simulink model "test"  (R2024b)
settings: Solver=ode4  StartTime=0.0  StopTime=2000  FixedStep=0.01  RelTol=1e-3
values from neighbouring files (symbols this model uses):
  g0 = 9.81    [llm_scenarios_case2.m]
  I_total = 0.5*(I_total + I_total.')    [total_inertia.m]    (also in total_inertia_backup.m = I_total + I_transformed)
undefined symbols (not defined in the file or in its folder): f_plant, GEOSAT, LLM, Mi, sigma_pos, sigma_vel, ST, Uoff, Uon
libraries: simulink x13, sharedTrackingLibrary x1
settings Model: Creator=simon  LastModifiedBy=simon
settings OptimizationCC: DefaultParameterBehavior=Inlined  EnhancedBackFolding=on  PassReuseOutputArgsAs=Individual arguments  ZeroExternalMemoryAtStartup=off  ZeroInternalMemoryAtStartup=off  MaxStackSize=64  OptimizeBlockOrder=speed  DifferentSizesBufferReuse=on  OptimizationCustomize=off  EfficientTunableParamExpr=on
settings DebuggingCC: ParameterTunabilityLossMsg=error
settings SFSimCC: MATLABDynamicMemAlloc=off
settings RTWCC: Description=Embedded Coder  SystemTargetFile=ert.tlc  HardwareBoard=Robot Operating System 2 (ROS 2)  TLCOptions="-aInlineSetEventsForThisBaseRateFcn=TLC_FALSE -aSuppressMultiTaskScheduler=TLC_FALSE  -aRateBasedStepFcn=0"  TemplateMakefile=ert_default_tmf  Toolchain=Colcon Tools  TargetLang=C++
settings CodeAppCC: ForceParamTrailComments=on  IgnoreCustomStorageClasses=off  OperatorAnnotations=on  SimulinkDataObjDesc=on  SFDataObjDesc=on  InsertBlockDesc=on
settings ERTTargetCC: CodeInterfacePackaging=C++ class  RootIOFormat=Structure reference

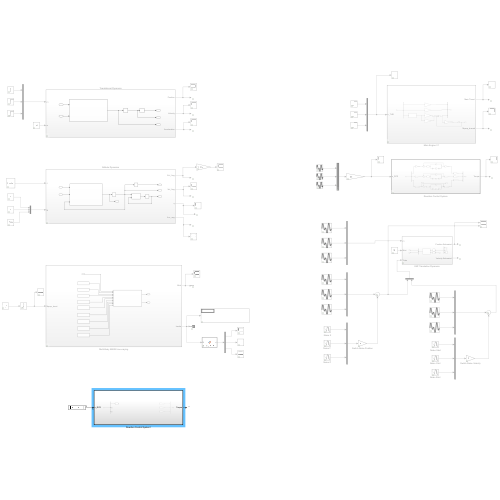
[thumbnail: Simulink's stored preview of the top-level diagram]
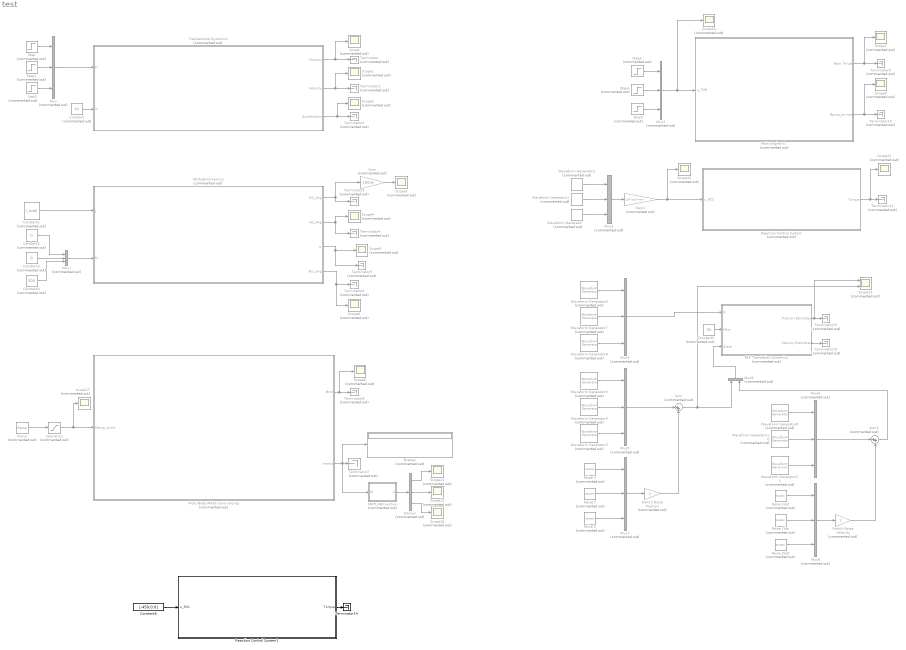
== system test ==
  " Noise X" : RandomNumber  Commented=on  Variance=sigma_pos^2  Seed=1  SampleTime=1/f_plant
  " Noise Xdot" : RandomNumber  Commented=on  Variance=sigma_vel^2  Seed=1  SampleTime=1/f_plant
  Attitude Dynamics : Subsystem  Commented=on
  Constant : Constant  Commented=on  Value=Mi
  Constant1 : Constant  Commented=on  Value=I_total
  Constant2 : Constant  Commented=on  Value=0
  Constant3 : Constant  Commented=on  Value=0
  Constant4 : Constant  Commented=on  Value=500
  Constant5 : Constant  Commented=on  Value=Mi
  Constant6 : Constant  Value=[-450;0;0]
  Demux : Demux  Commented=on  Outputs=3
  Display : Display  Commented=on
  EKF Translation Dynamics : Subsystem  Commented=on
  Gain : Gain  Commented=on  Gain=180/pi
  Gain1 : Gain  Commented=on  Gain=LLM.rcs.Fmax
  MATLAB Function : MATLAB Function  Commented=on  TreatAsAtomicUnit=on
  Main Engine V1 : Subsystem  Commented=on
  Multi-Body MASS time-varying : Subsystem  Commented=on
  Mux{,1..8} (9 alike) : Mux  Commented=on  Inputs=3
  Mux9 : Mux  Commented=on  Inputs=2
  Noise Y : RandomNumber  Commented=on  Variance=sigma_pos^2  Seed=2  SampleTime=1/f_plant
  Noise Ydot : RandomNumber  Commented=on  Variance=sigma_vel^2  Seed=2  SampleTime=1/f_plant
  Noise Z : RandomNumber  Commented=on  Variance=sigma_pos^2  Seed=3  SampleTime=1/f_plant
  Noise Zdot : RandomNumber  Commented=on  Variance=sigma_vel^2  Seed=3  SampleTime=1/f_plant
  Ramp : simulink/Sources/Ramp  Commented=on  slope=10  start=0  InitialOutput=0
  Reaction Control System : Subsystem  Commented=on  TreatAsAtomicUnit=on
  Reaction Control System1 : Subsystem  TreatAsAtomicUnit=on
  Saturation : Saturate  Commented=on  UpperLimit=0.01*LLM.propellant.mass  LowerLimit=0
  Scope{,1..12,14..17} (17 alike) : Scope  Commented=on
  Scope13 : Scope  Commented=on  NumInputPorts=2
  Step : Step  Commented=on  After=0  SampleTime=0
  Step1 : Step  Commented=on  After=0  SampleTime=0
  Step2 : Step  Commented=on  After=LLM.main_engine.Fmax  SampleTime=0
  Step3 : Step  Commented=on  Time=30  After=0.4  SampleTime=0
  Step4 : Step  Commented=on  Time=30  After=0.4  SampleTime=0
  Step5 : Step  Commented=on  Time=30  After=0.5  SampleTime=0
  Sum : Sum  Commented=on  Inputs=|++
  Sum1 : Sum  Commented=on  Inputs=|++
  Switch Noise Position : Gain  Commented=on
  Switch Noise Velocity : Gain  Commented=on
  Terminator{,1..13} (14 alike) : Terminator  Commented=on
  Terminator14 : Terminator
  Translational Dynamics : Subsystem  Commented=on
  Waveform Generator : simulink/Sources/Waveform Generator  Commented=on  OutMin=[]  OutMax=[]  OutDataTypeStr=double  SelectedSignal=1  Signals=sin('Amplitude', 1, 'Frequency', 0.3, 'Phase', 0)  BlockNames=MultiportSwitch_2c032cfd7e664ef  SampleTime=0.1
  Waveform Generator1 : simulink/Sources/Waveform Generator  Commented=on  OutMin=[]  OutMax=[]  OutDataTypeStr=double  SelectedSignal=1  Signals=sin('Amplitude', 1, 'Frequency', 0.3, 'Phase', 0)  BlockNames=MultiportSwitch_2c032cfd7e664ef  SampleTime=0.1
  Waveform Generator10 : simulink/Sources/Waveform Generator  Commented=on  OutMin=[]  OutMax=[]  OutDataTypeStr=double  SelectedSignal=1  Signals=cos(10, 1, 0)  BlockNames=MultiportSwitch_2c7686f9e0bf4b8  SampleTime=0.1
  Waveform Generator11 : simulink/Sources/Waveform Generator  Commented=on  OutMin=[]  OutMax=[]  OutDataTypeStr=double  SelectedSignal=1  Signals=cos(10, 1, 0)  BlockNames=MultiportSwitch_733c71b08a0b470  SampleTime=0.1
  Waveform Generator2 : simulink/Sources/Waveform Generator  Commented=on  OutMin=[]  OutMax=[]  OutDataTypeStr=double  SelectedSignal=1  Signals=sin('Amplitude', 1, 'Frequency', 0.3, 'Phase', 0)  BlockNames=MultiportSwitch_2c032cfd7e664ef  SampleTime=0.1
  Waveform Generator{3..8} (6 alike) : simulink/Sources/Waveform Generator  Commented=on  OutMin=[]  OutMax=[]  OutDataTypeStr=double  SelectedSignal=1  Signals=sin(10, 1, 0)  BlockNames=MultiportSwitch_61beab59be99459  SampleTime=0.1
  Waveform Generator9 : simulink/Sources/Waveform Generator  Commented=on  OutMin=[]  OutMax=[]  OutDataTypeStr=double  SelectedSignal=1  Signals=cos(10, 1, 0)  BlockNames=MultiportSwitch_701aef0e77f74ea  SampleTime=0.1
  wires:
  Mux/1 -> Translational Dynamics/1(FI)
  Constant/1 -> Translational Dynamics/2(m)
  Translational Dynamics/1(Position) -> Scope/1, Terminator/1
  Translational Dynamics/2(Velocity) -> Scope1/1, Terminator1/1
  Translational Dynamics/3(Acceleration) -> Scope2/1, Terminator2/1
  Step/1 -> Mux/1
  Step1/1 -> Mux/2
  Step2/1 -> Mux/3
  Attitude Dynamics/1(Eul_Ang) -> Gain/1, Terminator3/1
  Attitude Dynamics/2(Vel_Ang) -> Scope4/1, Terminator4/1
  Constant2/1 -> Mux1/1
  Constant3/1 -> Mux1/2
  Constant4/1 -> Mux1/3
  Mux1/1 -> Attitude Dynamics/2(M)
  Gain/1 -> Scope3/1
  Constant1/1 -> Attitude Dynamics/1(J)
  Attitude Dynamics/3(q) -> Scope5/1, Terminator5/1
  Attitude Dynamics/4(Acc_ang) -> Scope6/1, Terminator6/1
  Multi-Body MASS time-varying/1(Mtot) -> Terminator8/1, Scope8/1
  Ramp/1 -> Saturation/1
  Multi-Body MASS time-varying/2(Inertia) -> Display/1, Terminator7/1, MATLAB Function/1(M)
  Mux2/1 -> Scope10/1, Main Engine V1/1(u_THR)
  Step3/1 -> Mux2/1
  Step4/1 -> Mux2/2
  Step5/1 -> Mux2/3
  Main Engine V1/2(Mprop_burned) -> Scope9/1, Terminator10/1
  Main Engine V1/1("Main Thrust ") -> Scope7/1, Terminator9/1
  Gain1/1 -> Scope12/1, Reaction Control System/1(u_RCS)
  Reaction Control System/1(Torque) -> Scope11/1, Terminator11/1
  Waveform Generator2/1 -> Mux3/1
  Waveform Generator1/1 -> Mux3/2
  Mux3/1 -> Gain1/1
  Waveform Generator/1 -> Mux3/3
  Waveform Generator7/1 -> Mux4/2
  Waveform Generator6/1 -> Mux4/1
  Waveform Generator8/1 -> Mux4/3
  Waveform Generator3/1 -> Mux5/1
  Waveform Generator4/1 -> Mux5/2
  Waveform Generator5/1 -> Mux5/3
  Constant5/1 -> EKF Translation Dynamics/2(Mtot)
  Mux4/1 -> EKF Translation Dynamics/1(FI)
  EKF Translation Dynamics/1(Position Estimated) -> Scope13/1, Terminator12/1
  EKF Translation Dynamics/2(Velocity Estimated) -> Terminator13/1
  Waveform Generator10/1 -> Mux6/2
  Waveform Generator9/1 -> Mux6/1
  Waveform Generator11/1 -> Mux6/3
  " Noise Xdot"/1 -> Mux8/1
  Noise Y/1 -> Mux7/2
  Noise Ydot/1 -> Mux8/2
  Noise Zdot/1 -> Mux8/3
  " Noise X"/1 -> Mux7/1
  Noise Z/1 -> Mux7/3
  Mux8/1 -> Switch Noise Velocity/1
  Mux7/1 -> Switch Noise Position/1
  Mux5/1 -> Sum/1
  Switch Noise Position/1 -> Sum/2
  Mux6/1 -> Sum1/1
  Switch Noise Velocity/1 -> Sum1/2
  Sum/1 -> Mux9/1, Scope13/2
  Sum1/1 -> Mux9/2
  Mux9/1 -> EKF Translation Dynamics/3(State)
  MATLAB Function/1(d) -> Demux/1
  Demux/1 -> Scope14/1
  Demux/2 -> Scope15/1
  Demux/3 -> Scope16/1
  Saturation/1 -> Scope17/1, Multi-Body MASS time-varying/1(Mprop_burnt)
  Constant6/1 -> Reaction Control System1/1(u_RCS)
  Reaction Control System1/1(Torque) -> Terminator14/1

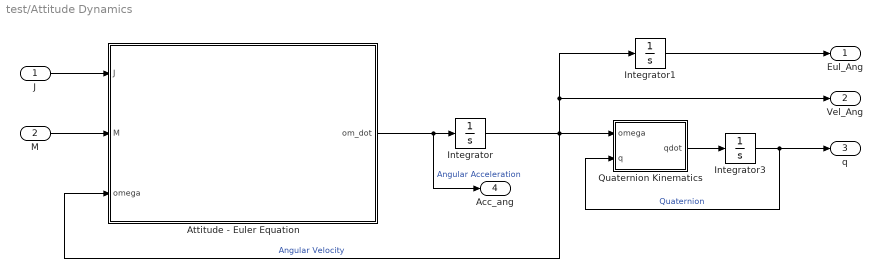
== system test/Attitude Dynamics ==
  J : Inport
  M : Inport  Port=2
  Attitude - Euler Equation : MATLAB Function  TreatAsAtomicUnit=on
  Integrator : Integrator  InitialCondition=[0;0;0]
  Integrator1 : Integrator  InitialCondition=[0;0;0]
  Integrator3 : Integrator  InitialCondition=[0;0;0;0]
  Quaternion Kinematics : MATLAB Function  TreatAsAtomicUnit=on
  Eul_Ang : Outport
  Vel_Ang : Outport  Port=2
  q : Outport  Port=3
  Acc_ang : Outport  Port=4
  wires:
  M/1 -> Attitude - Euler Equation/2(M)
  Attitude - Euler Equation/1(om_dot) -> Acc_ang/1, Integrator/1  "Angular Acceleration"
  Quaternion Kinematics/1(qdot) -> Integrator3/1
  Integrator/1 -> Vel_Ang/1, Integrator1/1, Attitude - Euler Equation/3(omega), Quaternion Kinematics/1(omega)  "Angular Velocity"
  Integrator3/1 -> q/1, Quaternion Kinematics/2(q)  "Quaternion"
  J/1 -> Attitude - Euler Equation/1(J)
  Integrator1/1 -> Eul_Ang/1

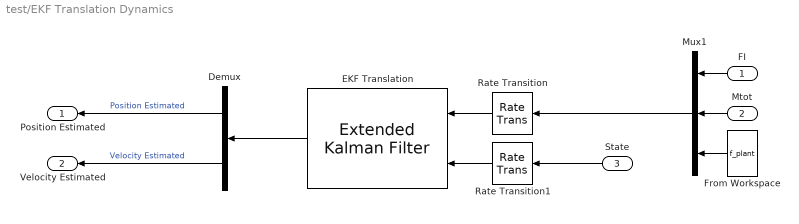
== system test/EKF Translation Dynamics ==
  FI : Inport
  Mtot : Inport  Port=2
  State : Inport  Port=3
  Demux : Demux  Outputs=2
  EKF Translation : sharedTrackingLibrary/Extended Kalman Filter  StateTransitionFcn=TranslationStateFcn  HasStateTransitionJacobianFcn=off  HasAdditiveProcessNoise=Additive  ProcessNoise=0.1  HasTimeVaryingProcessNoise=off  HasStateTransitionFcnExtraArgument=1  InitialState=0  InitialStateCovariance=1  MeasurementFcn1=TranslationMeasurementFcn  HasMeasurementJacobianFcn1=off  HasMeasurementEnablePort1=off  HasAdditiveMeasurementNoise1=Additive  MeasurementNoise1=1  HasTimeVaryingMeasurementNoise1=off  HasMeasurementFcnExtraArgument1=0  HasMeasurementWrapping1=off  MeasurementFcn2=myMeasurementFcn  HasMeasurementJacobianFcn2=off  HasMeasurementEnablePort2=off  HasAdditiveMeasurementNoise2=Additive  MeasurementNoise2=1  HasTimeVaryingMeasurementNoise2=off  HasMeasurementFcnExtraArgument2=0  HasMeasurementWrapping2=off  MeasurementFcn3=myMeasurementFcn  HasMeasurementJacobianFcn3=off  HasMeasurementEnablePort3=off  HasAdditiveMeasurementNoise3=Additive  MeasurementNoise3=1  HasTimeVaryingMeasurementNoise3=off  HasMeasurementFcnExtraArgument3=0  HasMeasurementWrapping3=off  MeasurementFcn4=myMeasurementFcn  HasMeasurementJacobianFcn4=off  HasMeasurementEnablePort4=off  HasAdditiveMeasurementNoise4=Additive  MeasurementNoise4=1  HasTimeVaryingMeasurementNoise4=off  HasMeasurementFcnExtraArgument4=0  HasMeasurementWrapping4=off  MeasurementFcn5=myMeasurementFcn  HasMeasurementJacobianFcn5=off  HasMeasurementEnablePort5=off  HasAdditiveMeasurementNoise5=Additive  MeasurementNoise5=1  HasTimeVaryingMeasurementNoise5=off  HasMeasurementFcnExtraArgument5=0  HasMeasurementWrapping5=off  EnableMultirate=off  StateTransitionFcnSampleTime=1  MeasurementFcn1SampleTime=1  MeasurementFcn2SampleTime=1  MeasurementFcn3SampleTime=1  MeasurementFcn4SampleTime=1  MeasurementFcn5SampleTime=1  UseCurrentEstimator=on  OutputStateCovariance=off  DataType=double  SampleTime=1/f_plant  NumberOfMeasurements=1
  From Workspace : FromWorkspace  VariableName=f_plant
  Mux1 : Mux  Inputs=3
  Rate Transition : RateTransition  OutPortSampleTime=1/f_plant
  Rate Transition1 : RateTransition  OutPortSampleTime=1/f_plant
  Position Estimated : Outport
  Velocity Estimated : Outport  Port=2
  wires:
  State/1 -> Rate Transition1/1
  Rate Transition1/1 -> EKF Translation/2
  FI/1 -> Mux1/1
  From Workspace/1 -> Mux1/3
  Mtot/1 -> Mux1/2
  EKF Translation/1 -> Demux/1
  Mux1/1 -> Rate Transition/1
  Rate Transition/1 -> EKF Translation/1
  Demux/2 -> Velocity Estimated/1  "Velocity Estimated"
  Demux/1 -> Position Estimated/1  "Position Estimated"

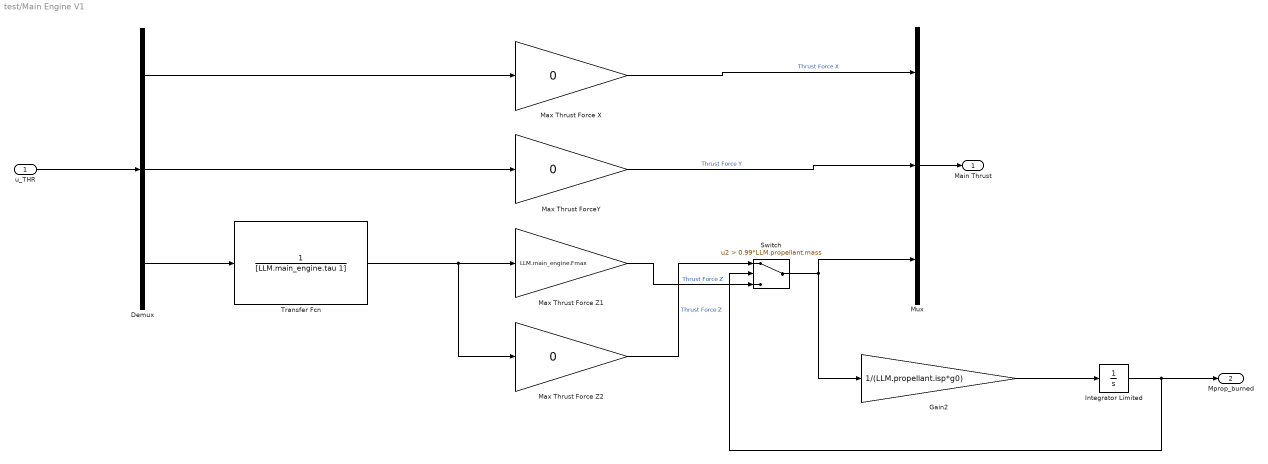
== system test/Main Engine V1 ==
  u_THR : Inport
  Demux : Demux  Outputs=3
  Gain2 : Gain  Gain=1/(LLM.propellant.isp*g0)
  Integrator Limited : Integrator  LimitOutput=on  UpperSaturationLimit=LLM.propellant.mass  LowerSaturationLimit=0
  Max Thrust Force X : Gain  Gain=0
  Max Thrust Force Z1 : Gain  Gain=LLM.main_engine.Fmax
  Max Thrust Force Z2 : Gain  Gain=0
  Max Thrust ForceY : Gain  Gain=0
  Mux : Mux  Inputs=3
  Switch : Switch  Criteria=u2 > Threshold  Threshold=0.99*LLM.propellant.mass  SaturateOnIntegerOverflow=off  InputSameDT=off
  Transfer Fcn : TransferFcn  Denominator=[LLM.main_engine.tau 1]
  "Main Thrust " : Outport
  Mprop_burned : Outport  Port=2
  wires:
  Transfer Fcn/1 -> Max Thrust Force Z2/1, Max Thrust Force Z1/1
  Mux/1 -> "Main Thrust "/1
  Demux/3 -> Transfer Fcn/1
  Max Thrust Force X/1 -> Mux/1  "Thrust Force X"
  Max Thrust ForceY/1 -> Mux/2  "Thrust Force Y"
  u_THR/1 -> Demux/1
  Demux/1 -> Max Thrust Force X/1
  Demux/2 -> Max Thrust ForceY/1
  Gain2/1 -> Integrator Limited/1
  Integrator Limited/1 -> Mprop_burned/1, Switch/2
  Switch/1 -> Gain2/1, Mux/3
  Max Thrust Force Z2/1 -> Switch/1  "Thrust Force Z"
  Max Thrust Force Z1/1 -> Switch/3  "Thrust Force Z"

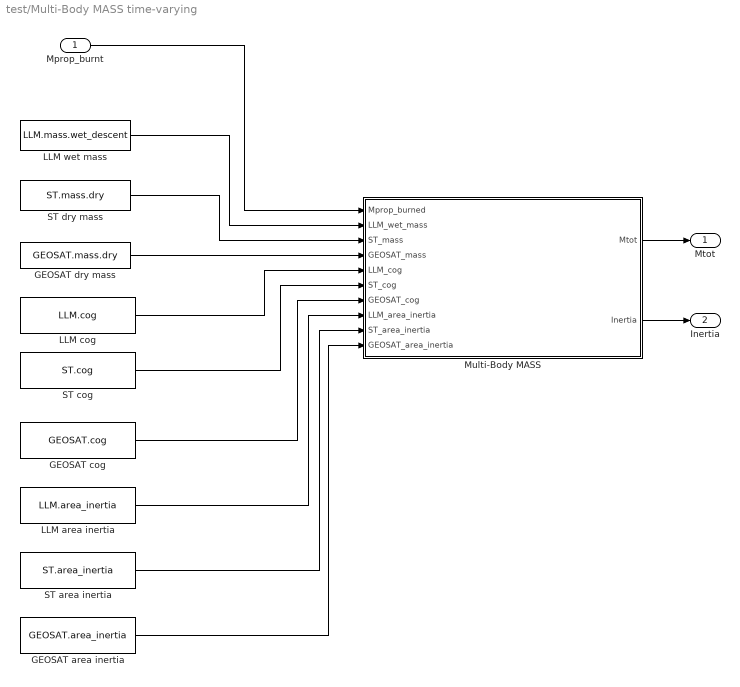
== system test/Multi-Body MASS time-varying ==
  Mprop_burnt : Inport  OutDataTypeStr=double
  GEOSAT area inertia : Constant  Value=GEOSAT.area_inertia
  GEOSAT cog : Constant  Value=GEOSAT.cog
  GEOSAT dry mass : Constant  Value=GEOSAT.mass.dry
  LLM area inertia : Constant  Value=LLM.area_inertia
  LLM cog : Constant  Value=LLM.cog
  LLM wet mass : Constant  Value=LLM.mass.wet_descent
  Multi-Body MASS : MATLAB Function  TreatAsAtomicUnit=on
  ST area inertia : Constant  Value=ST.area_inertia
  ST cog : Constant  Value=ST.cog
  ST dry mass : Constant  Value=ST.mass.dry
  Mtot : Outport
  Inertia : Outport  Port=2
  wires:
  LLM wet mass/1 -> Multi-Body MASS/2(LLM_wet_mass)
  GEOSAT area inertia/1 -> Multi-Body MASS/10(GEOSAT_area_inertia)
  LLM cog/1 -> Multi-Body MASS/5(LLM_cog)
  GEOSAT dry mass/1 -> Multi-Body MASS/4(GEOSAT_mass)
  ST area inertia/1 -> Multi-Body MASS/9(ST_area_inertia)
  ST dry mass/1 -> Multi-Body MASS/3(ST_mass)
  GEOSAT cog/1 -> Multi-Body MASS/7(GEOSAT_cog)
  LLM area inertia/1 -> Multi-Body MASS/8(LLM_area_inertia)
  Multi-Body MASS/2(Inertia) -> Inertia/1
  Mprop_burnt/1 -> Multi-Body MASS/1(Mprop_burned)
  Multi-Body MASS/1(Mtot) -> Mtot/1
  ST cog/1 -> Multi-Body MASS/6(ST_cog)

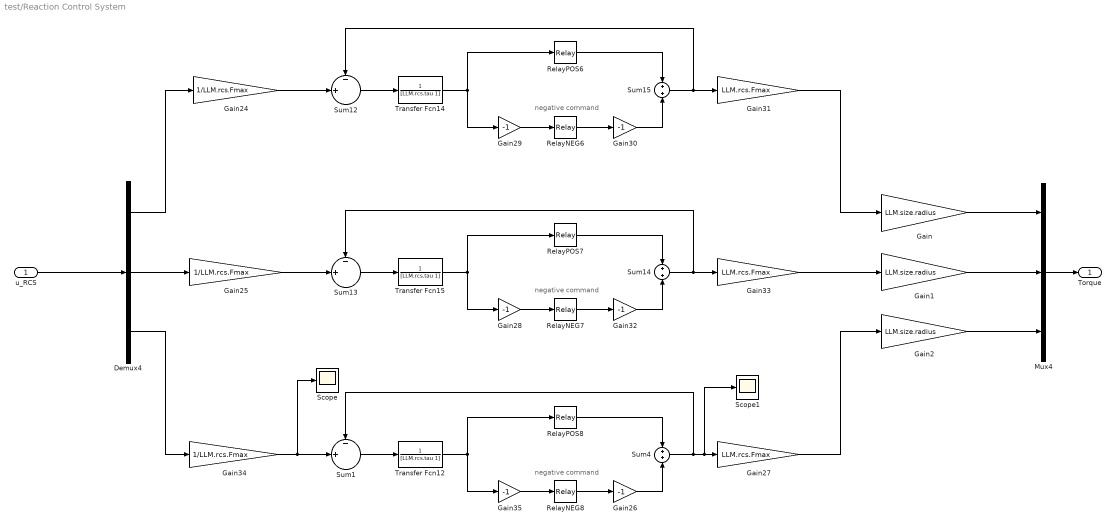
== system test/Reaction Control System ==
  note: negative command
  note: negative command
  note: negative command
  u_RCS : Inport
  Demux4 : Demux  Outputs=3
  Gain : Gain  Gain=LLM.size.radius
  Gain1 : Gain  Gain=LLM.size.radius
  Gain2 : Gain  Gain=LLM.size.radius
  Gain24 : Gain  Gain=1/LLM.rcs.Fmax
  Gain25 : Gain  Gain=1/LLM.rcs.Fmax
  Gain{26,28..30,32,35} (6 alike) : Gain  Gain=-1
  Gain27 : Gain  Gain=LLM.rcs.Fmax
  Gain31 : Gain  Gain=LLM.rcs.Fmax
  Gain33 : Gain  Gain=LLM.rcs.Fmax
  Gain34 : Gain  Gain=1/LLM.rcs.Fmax
  Mux4 : Mux  Inputs=3
  RelayNEG6 : Relay  OnSwitchValue=Uon  OffSwitchValue=Uoff
  RelayNEG7 : Relay  OnSwitchValue=Uon  OffSwitchValue=Uoff
  RelayNEG8 : Relay  OnSwitchValue=Uon  OffSwitchValue=Uoff
  RelayPOS6 : Relay  OnSwitchValue=Uon  OffSwitchValue=Uoff
  RelayPOS7 : Relay  OnSwitchValue=Uon  OffSwitchValue=Uoff
  RelayPOS8 : Relay  OnSwitchValue=Uon  OffSwitchValue=Uoff
  Scope : Scope
  Scope1 : Scope
  Sum1 : Sum  Inputs=-||+|||
  Sum12 : Sum  Inputs=-||+|||
  Sum13 : Sum  Inputs=-||+|||
  Sum14 : Sum  Inputs=+|+
  Sum15 : Sum  Inputs=+|+
  Sum4 : Sum  Inputs=+|+
  Transfer Fcn12 : TransferFcn  Numerator=1  Denominator=[LLM.rcs.tau 1]
  Transfer Fcn14 : TransferFcn  Numerator=1  Denominator=[LLM.rcs.tau 1]
  Transfer Fcn15 : TransferFcn  Numerator=1  Denominator=[LLM.rcs.tau 1]
  Torque : Outport
  wires:
  RelayNEG7/1 -> Gain32/1
  RelayNEG8/1 -> Gain26/1
  RelayPOS7/1 -> Sum14/1
  Gain27/1 -> Gain2/1
  Sum4/1 -> Scope1/1, Gain27/1, Sum1/1
  RelayPOS6/1 -> Sum15/1
  Gain24/1 -> Sum12/2
  Gain30/1 -> Sum15/2
  Transfer Fcn12/1 -> Gain35/1, RelayPOS8/1
  Gain26/1 -> Sum4/2
  Sum1/1 -> Transfer Fcn12/1
  Transfer Fcn15/1 -> Gain28/1, RelayPOS7/1
  RelayPOS8/1 -> Sum4/1
  Demux4/3 -> Gain34/1
  RelayNEG6/1 -> Gain30/1
  Gain28/1 -> RelayNEG7/1
  Demux4/1 -> Gain24/1
  Sum15/1 -> Gain31/1, Sum12/1
  Gain25/1 -> Sum13/2
  Gain32/1 -> Sum14/2
  Gain31/1 -> Gain/1
  Sum13/1 -> Transfer Fcn15/1
  Demux4/2 -> Gain25/1
  Sum14/1 -> Gain33/1, Sum13/1
  Gain33/1 -> Gain1/1
  Gain35/1 -> RelayNEG8/1
  Gain29/1 -> RelayNEG6/1
  Sum12/1 -> Transfer Fcn14/1
  Transfer Fcn14/1 -> Gain29/1, RelayPOS6/1
  u_RCS/1 -> Demux4/1
  Mux4/1 -> Torque/1
  Gain/1 -> Mux4/1
  Gain1/1 -> Mux4/2
  Gain2/1 -> Mux4/3
  Gain34/1 -> Scope/1, Sum1/2

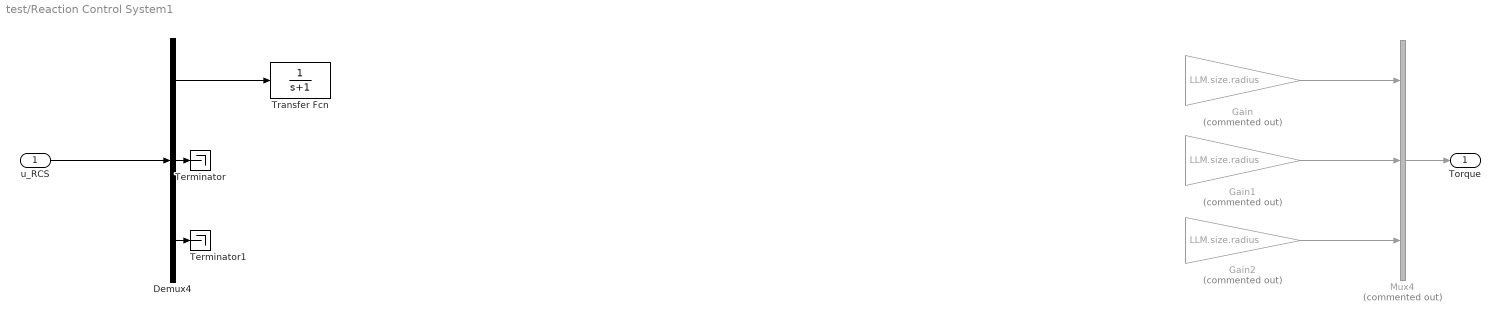
== system test/Reaction Control System1 ==
  u_RCS : Inport
  Demux4 : Demux  Outputs=3
  Gain : Gain  Commented=on  Gain=LLM.size.radius
  Gain1 : Gain  Commented=on  Gain=LLM.size.radius
  Gain2 : Gain  Commented=on  Gain=LLM.size.radius
  Mux4 : Mux  Commented=on  Inputs=3
  Terminator : Terminator
  Terminator1 : Terminator
  Transfer Fcn : TransferFcn  Denominator=[1 1]
  Torque : Outport
  wires:
  u_RCS/1 -> Demux4/1
  Mux4/1 -> Torque/1
  Gain/1 -> Mux4/1
  Gain1/1 -> Mux4/2
  Gain2/1 -> Mux4/3
  Demux4/2 -> Terminator/1
  Demux4/3 -> Terminator1/1
  Demux4/1 -> Transfer Fcn/1

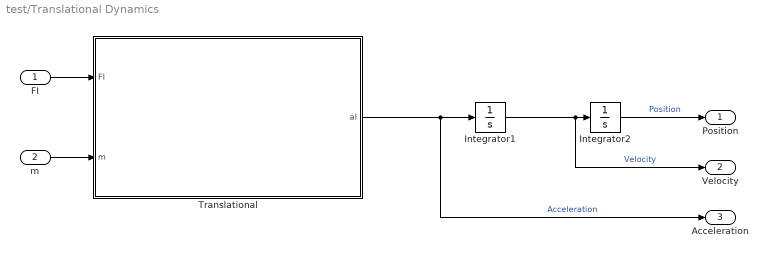
== system test/Translational Dynamics ==
  FI : Inport
  m : Inport  Port=2
  Integrator1 : Integrator
  Integrator2 : Integrator
  Translational : MATLAB Function  TreatAsAtomicUnit=on
  Position : Outport
  Velocity : Outport  Port=2
  Acceleration : Outport  Port=3
  wires:
  Integrator1/1 -> Velocity/1, Integrator2/1  "Velocity"
  Integrator2/1 -> Position/1  "Position"
  FI/1 -> Translational/1(FI)
  Translational/1(aI) -> Acceleration/1, Integrator1/1  "Acceleration"
  m/1 -> Translational/2(m)

== matlab function test/Attitude Dynamics/Attitude - Euler Equation ==
  data: J input; om_dot output; M input; omega input
function om_dot = Rot_3D(J, M, omega)
om_dot = inv(J)*(M-cross(omega,(J*omega)));

== matlab function test/Translational Dynamics/Translational ==
  data: FI input; aI output; m input
function aI = Acc_3D(FI, m)
% --- INPUT ---
% FI    : 3x1 force in inertial frame [N]
% m     : mass [kg]

% --- OUTPUT ---
% aI    : acceleration in inertial frame [m/s^2]

% lunar gravity in inertial frame (verso -Z)
gL = 1.622;
gI = [0; 0; -gL];

%  Acceleration
aI = FI./m + gI;
end




% Matrice di rotazione body -> inerziale (ZYX: Rz * Ry * Rx)
% roll = eul_ang(1);
% pitch = eul_ang(2);
% yaw = eul_ang(3);
% 
% cY = cos(yaw);   sY = sin(yaw);
% cP = cos(pitch); sP = sin(pitch);
% cR = cos(roll);  sR = sin(roll);
% 
% Rz = [ cY -sY  0;
%        sY  cY  0;
%         0   0  1];
% 
% Ry = [ cP  0  sP;
%         0  1   0;
%       -sP  0  cP];
% 
% Rx = [ 1   0   0;
%        0  cR -sR;
%        0  sR  cR];
% 
% R_IB = Rz * Ry * Rx;      % ruota dal body all'inerziale
% 
% % Forza in inerziale e seconda legge di Newton
% FI = R_IB * FB;

== matlab function test/MATLAB Function ==
  data: M input; d output
function d = diag_extract(M)
%#codegen
d = diag(M);

== matlab function test/Multi-Body MASS time-varying/Multi-Body MASS ==
  data: Mprop_burned input; Mtot output; Inertia output; LLM_wet_mass input; ST_mass input; GEOSAT_mass input; LLM_cog input; ST_cog input; GEOSAT_cog input; LLM_area_inertia input size=[3 3]; ST_area_inertia input size=[3 3]; GEOSAT_area_inertia input size=[3 3]
function [Mtot, Inertia] = fcn(Mprop_burned, LLM_wet_mass, ST_mass, GEOSAT_mass, LLM_cog, ST_cog, GEOSAT_cog, LLM_area_inertia, ST_area_inertia, GEOSAT_area_inertia)
% --- INPUT ---
% Mprop_burned : total propellant burned so far
% LLM_wet_mass : total LLM mass (dry = full propellant)
% ST_mass : Space Tug mass (dry)
% GEOSAT_mass : GEOSAT mass (dry)
% LLM_cog : LLM center of gravity 3x1
% ST_cog : ST center of gravity 3x1
% GEOSAT_cog : GEOSAT center of gravity 3x1

% --- OUTPUT --- 
% Mtot : Total mass of the multi-body system
% Inertia : Inertia Matrix

%% === CENTER OF MASSES (corretto) ===
% Assicurati che i CoG siano colonne 3x1
LLM_cog    = LLM_cog(:);
ST_cog     = ST_cog(:);
GEOSAT_cog = GEOSAT_cog(:);

% Massa istantanea del LLM
LLM_mass = LLM_wet_mass - Mprop_burned;

% (Se non già definiti) masse costanti degli altri due
% ST_mass e GEOSAT_mass devono essere scalar già nel workspace

% Massa totale
Mtot = LLM_mass + ST_mass + GEOSAT_mass;

% Centro di massa totale (posizione, non pesata)
COMtot = (LLM_mass*LLM_cog + ST_mass*ST_cog + GEOSAT_mass*GEOSAT_cog) / Mtot;

%% === INERTIA OF MULTI-BODY SYSTEM (corretto) ===
% Vettori spostamento dal CoM totale (posizioni pure)
r_LLM    = LLM_cog    - COMtot;   % 3x1
r_ST     = ST_cog     - COMtot;   % 3x1
r_GEOSAT = GEOSAT_cog - COMtot;   % 3x1

% Tensori centroidali (scalano con la massa a geometria fissa)
I_LLM_c    = LLM_mass    * LLM_area_inertia;     % 3x3
I_ST_c     = ST_mass     * ST_area_inertia;      % 3x3
I_GEOSAT_c = GEOSAT_mass * GEOSAT_area_inertia;  % 3x3

% Teorema degli assi paralleli (forma tensoriale)
parallel = @(m,r) m * ( (r.'*r)*eye(3) - (r*r.') );

Inertia = I_LLM_c    + parallel(LLM_mass,    r_LLM) ...
        + I_ST_c     + parallel(ST_mass,     r_ST)  ...
        + I_GEOSAT_c + parallel(GEOSAT_mass, r_GEOSAT);

% Simmetrizzazione numerica (consigliata)
Inertia = 0.5*(Inertia + Inertia.');

== matlab function test/Attitude Dynamics/Quaternion Kinematics ==
  data: omega input; qdot output; q input
function qdot = fcn(omega,q)

Omega = [0 -omega(1) -omega(2) -omega(3);
         omega(1) 0 omega(3) omega(2);
         omega(2) omega(3) 0 omega(1);
         omega(3) omega(2) omega(1) 0];

q0 = q(1);
q1 = q(2);
q2 = q(3);
q3 = q(4);

qdot = 0.5*Omega*[q0 q1 q2 q3]';
